simulink model "UAV_model"  (R2023a)
settings: Solver=VariableStepAuto  StartTime=0.0  StopTime=10.0  RelTol=1e-3
undefined symbols (not defined in the file): Dt, Fb, Fd, g, I, m, R, taub
libraries: aerolibutil x2, Contact_Forces_Lib x1
settings Model: Creator=dcest  LastModifiedBy=jonas
settings OptimizationCC: ReuseModelBlockBuffer=off

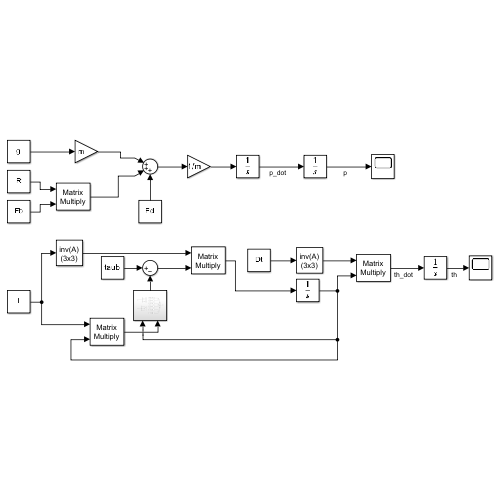
[thumbnail: Simulink's stored preview of the top-level diagram]
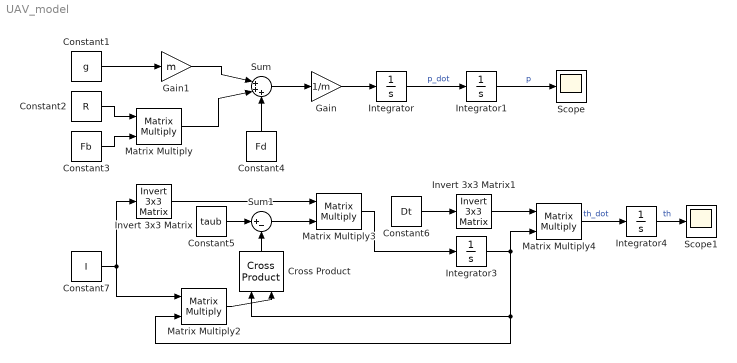
== system UAV_model ==
  Constant1 : Constant  Value=g
  Constant2 : Constant  Value=R
  Constant3 : Constant  Value=Fb
  Constant4 : Constant  Value=Fd
  Constant5 : Constant  Value=taub
  Constant6 : Constant  Value=Dt
  Constant7 : Constant  Value=I
  Cross Product : Contact_Forces_Lib/Math/Cross Product  SystemSampleTime=-1  VariantActivationTime=update diagram  Latency=0  AutoFrameSizeCalculation=off
      settings: SourceProductName=Simscape Multibody Contact Forces Library
  Gain : Gain  Gain=1/m
  Gain1 : Gain  Gain=m
  Integrator{,1,3..4} (4 alike) : Integrator
  Invert 3x3 Matrix : aerolibutil/Invert  3x3 Matrix
  Invert 3x3 Matrix1 : aerolibutil/Invert  3x3 Matrix
  Matrix Multiply{,2..4} (4 alike) : Product  Multiplication=Matrix(*)
  Scope : Scope
  Scope1 : Scope
  Sum : Sum  Inputs=|+++
  Sum1 : Sum  Inputs=|+-
  wires:
  Constant2/1 -> Matrix Multiply/1
  Constant3/1 -> Matrix Multiply/2
  Matrix Multiply/1 -> Sum/2
  Constant4/1 -> Sum/3
  Sum/1 -> Gain/1
  Gain/1 -> Integrator/1
  Constant7/1 -> Matrix Multiply2/1, Invert 3x3 Matrix/1
  Matrix Multiply2/1 -> Cross Product/2
  Constant5/1 -> Sum1/1
  Cross Product/1 -> Sum1/2
  Invert 3x3 Matrix/1 -> Matrix Multiply3/1
  Sum1/1 -> Matrix Multiply3/2
  Matrix Multiply3/1 -> Integrator3/1
  Integrator3/1 -> Matrix Multiply2/2, Cross Product/1, Matrix Multiply4/2
  Constant6/1 -> Invert 3x3 Matrix1/1
  Invert 3x3 Matrix1/1 -> Matrix Multiply4/1
  Constant1/1 -> Gain1/1
  Gain1/1 -> Sum/1
  Integrator1/1 -> Scope/1  "p"
  Integrator/1 -> Integrator1/1  "p_dot"
  Matrix Multiply4/1 -> Integrator4/1  "th_dot"
  Integrator4/1 -> Scope1/1  "th"
